simulink model "SSMC"  (R2026b)
settings Model: Creator=Yahoff  LastModifiedBy=Yahoff

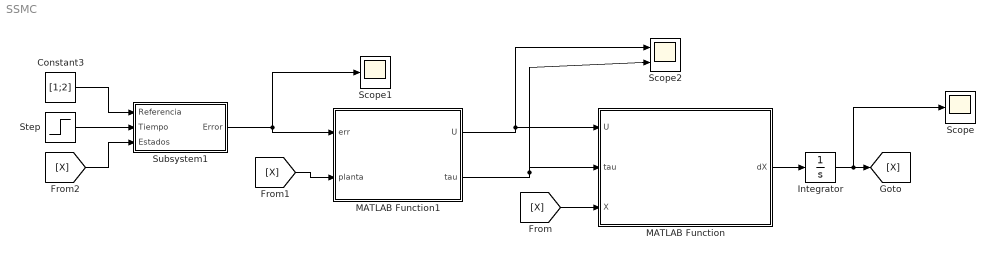
== system SSMC ==
  Constant3 : Constant  Value=[1;2]
  Integrator : Integrator  InitialCondition=[0;0;0;0;0;0]
  MATLAB Function : MATLAB Function  TreatAsAtomicUnit=on
  MATLAB Function1 : MATLAB Function  TreatAsAtomicUnit=on
  Scope : Scope
      settings: ActiveDisplayYMinimum=-0.25952515172247687  ActiveDisplayYMaximum=2.3357263655022922
  Scope1 : Scope
      settings: ActiveDisplayYMinimum=-0.13405317784249143  ActiveDisplayYMaximum=0.41916600704598622
  Scope2 : Scope  NumInputPorts=2
      settings: ActiveDisplayYMinimum=-674.86732252349577  ActiveDisplayYMaximum=90.487033234979336  DataLoggingVariableName=ScopeData2
  Step : Step  SampleTime=0
  Subsystem1 : Subsystem
  wires:
  MATLAB Function/1(dX) -> Integrator/1
  Integrator/1 -> Scope/1, [X]
  [X] -> MATLAB Function/3(X)
  [X] -> MATLAB Function1/2(planta)
  MATLAB Function1/1(U) -> Scope2/1, MATLAB Function/1(U)
  MATLAB Function1/2(tau) -> Scope2/2, MATLAB Function/2(tau)
  [X] -> Subsystem1/3(Estados)
  Constant3/1 -> Subsystem1/1(Referencia)
  Step/1 -> Subsystem1/2(Tiempo)
  Subsystem1/1(Error) -> Scope1/1, MATLAB Function1/1(err)

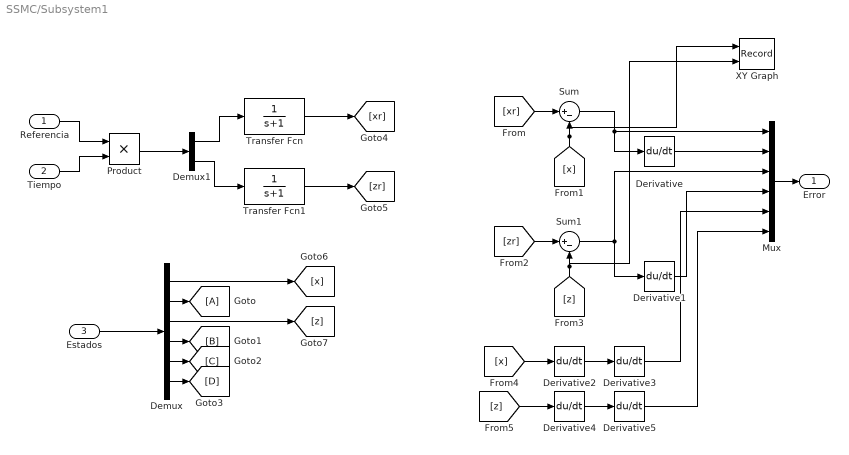
== system SSMC/Subsystem1 ==
  Referencia : Inport
  Tiempo : Inport  Port=2
  Estados : Inport  Port=3
  Demux : Demux  Outputs=6
  Demux1 : Demux  Outputs=2
  Derivative{,1..5} (6 alike) : Derivative
  Goto : Goto
  Mux : Mux  Inputs=6
  Product : Product
  Sum : Sum  Inputs=|+-
  Sum1 : Sum  Inputs=|+-
  Transfer Fcn : TransferFcn  Denominator=[1 1]
  Transfer Fcn1 : TransferFcn  Denominator=[1 1]
  XY Graph : Record  NumPorts=2.0  FileSettingsInternal="{\"entries\":[{\"content\":{\"excelSettings\":{\"content\":{},\"type\":\"Streamout.ExcelSettings\"},\"parquetSettings\":{\"content\":{},\"type\":\"Streamout.ParquetSettings\"}},\"type\":\"Streamout.FileSettingStorage\",\"uuid\":\"\"}],\"packageUris\":[\"http:\\/\\/schema.mathworks.com\\/mf0\\/streamout_blocks\\/R2020a\"],\"version\":\"1.0\"}"  FrameSettings=[0, 0]  Layout=[1 1]  SignalsInternal="{\"entries\":[{\"content\":{\"signals\":[{\"content\":{\"blockPath\":[],\"dimensions\":[1],\"domain\":\"\",\"lineColor\":\"#a2142f\",\"plots\":[ 1 ],\"port\":1,\"sid\":[\"\"],\"signalID\":1,\"signalName\":\"From1\"},\"type\":\"RecordBlkView.Signal\",\"uuid\":\"\"},{\"content\":{\"blockPath\":[],\"dimensions\":[1],\"domain\":\"\",\"lineColor\":\"#139fff\",\"plots\":[ 1 ],\"port\":2,\"sid\":[\"\"],\"signalID\":2,\"signalName\":\"From3\"},\"type\":\"RecordBlkView.Signal\",\"uuid\":\"\"}]},\"type\":\"RecordBlkView.InputSignals\",\"uuid\":\"\"}],\"packageUris\":[\"http:\\/\\/schema.mathworks.com\\/mf0\\/streamout_blocks\\/R2020a\"],\"version\":\"1.0\"}"  VisualizationBindings="{\"xyplotplugin\":{\"info\":[{\"series\":[{\"bindingParametersList\":[{\"parameter\":\"X-Axis\",\"signalID\":1,\"signalName\":\"From1\"},{\"parameter\":\"Y-Axis\",\"signalID\":2,\"signalName\":\"From3\"}],\"seriesID\":0}],\"subplotID\":1}]}}"  CompatibilityTag=XY
  Error : Outport
  wires:
  Demux/3 -> [z]
  Demux/1 -> [x]
  Demux/5 -> [C]
  Demux/6 -> [D]
  Estados/1 -> Demux/1
  Demux/2 -> Goto/1
  Demux/4 -> [B]
  Referencia/1 -> Product/1
  Tiempo/1 -> Product/2
  Product/1 -> Demux1/1
  Demux1/2 -> Transfer Fcn1/1
  Demux1/1 -> Transfer Fcn/1
  Transfer Fcn/1 -> [xr]
  Transfer Fcn1/1 -> [zr]
  [xr] -> Sum/1
  [x] -> XY Graph/1, Sum/2
  [zr] -> Sum1/1
  [z] -> XY Graph/2, Sum1/2
  Sum/1 -> Derivative/1, Mux/1
  Sum1/1 -> Mux/3, Derivative1/1
  Derivative/1 -> Mux/2
  Derivative1/1 -> Mux/4
  Mux/1 -> Error/1
  Derivative2/1 -> Derivative3/1
  Derivative4/1 -> Derivative5/1
  [x] -> Derivative2/1
  [z] -> Derivative4/1
  Derivative3/1 -> Mux/5
  Derivative5/1 -> Mux/6

== matlab function SSMC/MATLAB Function1 ==
  data: err input; U output; planta input; tau output
function [U, tau] = control(err, planta)

    m = 1; g = 9.81;
    kth = 100; kom =50;

    k=4;%4
    m=1;%1
    l=2;%2
    n=1;%1

    ex = err(1);
    dex = err(2);
    ez = err(3);   
    dez = err(4);
    xrdd=err(5);
    zrdd=err(6);

    x     = planta(1);
    xdot  = planta(2);
    z     = planta(3);
    zdot  = planta(4);
    th    = planta(5);
    thdot = planta(6);

    sx = dex + n*ex;
    vx = -n*ex + l*sat(sx);
   
    sz = dez + m*ez;
    vz = -m*ez + k*sat(sz);

    U   = m*sqrt(vx^2 + (vz+g)^2);
    thd = atan2(-vx, vz+g);

    e = th - thd;
    de = thdot;

    j = 2000;
    b = 10;

    s = de +  b*e;
    tau = - b*de - j*sat(s);

    %tau = -kth*(th - thd) - kom*thdot;
end



function y = sat(u)
if u > 1
    y = 1;
elseif u < -1
    y = -1;
else
    y = u;
end
end

== matlab function SSMC/MATLAB Function ==
  data: U input; dX output; tau input; X input
function dX = planta(U, tau, X)

    m = 1; J = 1; g = 9.81;
    kth = 30; kom = 12;

    x     = X(1);
    xdot  = X(2);
    z     = X(3);
    zdot  = X(4);
    th    = X(5);
    thdot = X(6);

    xdd  = -(U/m)*sin(th);
    zdd  =  (U/m)*cos(th) - g;
    thdd =  tau/J;

    dX = [xdot; xdd; zdot; zdd; thdot; thdd];
